simulink model "pam_system"  (R2024b)
settings: Solver=VariableStepAuto  StartTime=0.0  StopTime=1  RelTol=1e-3
model workspace (MAT data in the model file):
  bit_interval = 0.01
  carrier_interval = 0.001
  reference_energy = 0.005
  sampling_interval = 0.0001
undefined symbols (not defined in the file or in its folder): DiscIntNeverNeededParam
libraries: commchan3 x1, commrandsrc3 x1
settings Model: Creator=YN53IX  LastModifiedBy=rasm2
settings SolverCC: AlgebraicLoopSolver=TrustRegion
settings DebuggingCC: ArithmeticOperatorsInVariantConditions=warning
settings SFSimCC: CustomCodeUndefinedFunction=UseInterfaceOnly
settings RTWCC: GPUComputeCapability=3.5

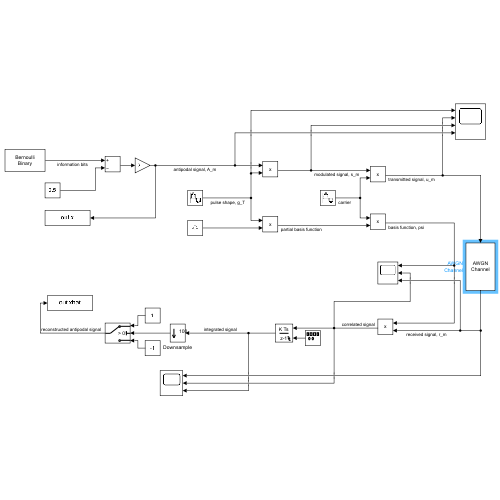
[thumbnail: Simulink's stored preview of the top-level diagram]
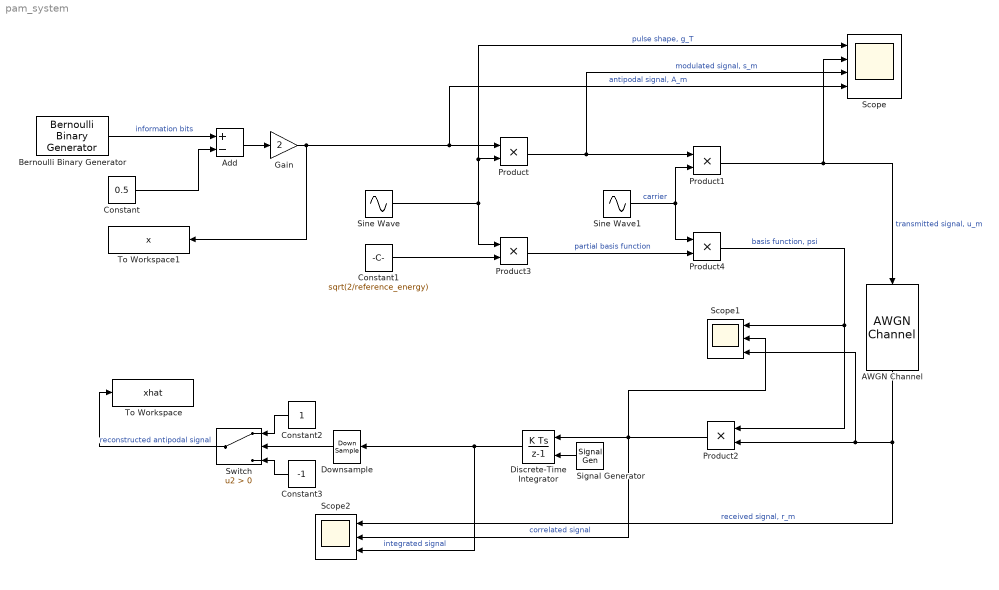
== system pam_system ==
  AWGN Channel : commchan3/AWGN Channel  LegacyMode=on  NoiseMethod="Signal to noise ratio  (SNR)"  noiseMode="Signal to noise ratio  (SNR)"  EbNo=0  EsNo=10  SNR=-10  BitsPerSymbol=1  SignalPower=1  SamplesPerSymbol=1  SymbolPeriod=(1.000000e-04 * 1)  VarianceSource=Parameter  Variance=1  RandomStream=Global stream  Seed=42  SimulateUsing=Code generation
  Add : Sum  Inputs=+-
  Bernoulli Binary Generator : commrandsrc3/Bernoulli Binary Generator  ProbabilityOfZero=0.5  SeedSource=Parameter  Seed=42  SampleTime=bit_interval  SamplesPerFrame=1  OutputDataType=double  SimulateUsing=Interpreted execution
  Constant : Constant  Value=0.5
  Constant1 : Constant  Value=sqrt(2/reference_energy)
  Constant2 : Constant
  Constant3 : Constant  Value=-1
  Discrete-Time Integrator : DiscreteIntegrator  ExternalReset=falling  SampleTime=sampling_interval  ICPrevOutput=DiscIntNeverNeededParam  ICPrevScaledInput=DiscIntNeverNeededParam
  Downsample : DownSample  N=100  phase=99  RateOptions=Allow multirate processing
  Gain : Gain  Gain=2
  Product{,1..4} (5 alike) : Product
  Scope : Scope  NumInputPorts=4
  Scope1 : Scope  NumInputPorts=3
  Scope2 : Scope  NumInputPorts=3
  Signal Generator : SignalGenerator  WaveForm=square  Frequency=1/bit_interval
  Sine Wave : Sin  Frequency=2*pi / bit_interval  Phase=pi/2  SampleTime=sampling_interval
  Sine Wave1 : Sin  Frequency=2 * pi / carrier_interval  Phase=pi/2  SampleTime=sampling_interval
  Switch : Switch  Criteria=u2 > Threshold  SaturateOnIntegerOverflow=off  InputSameDT=off
  To Workspace : ToWorkspace  VariableName=xhat  SampleTime=-1
      settings: Save2DSignal=2-D array (concatenate along first dimension)
  To Workspace1 : ToWorkspace  VariableName=x  SampleTime=-1
      settings: Save2DSignal=2-D array (concatenate along first dimension)
  wires:
  Bernoulli Binary Generator/1 -> Add/1  "information bits"
  Constant/1 -> Add/2
  Add/1 -> Gain/1
  Gain/1 -> To Workspace1/1, Scope/4, Product/1  "antipodal signal, A_m"
  Sine Wave/1 -> Scope/1, Product/2, Product3/1  "pulse shape, g_T"
  Product/1 -> Scope/3, Product1/1  "modulated signal, s_m"
  Sine Wave1/1 -> Product1/2, Product4/1  "carrier"
  Product1/1 -> Scope/2, AWGN Channel/1  "transmitted signal, u_m"
  AWGN Channel/1 -> Scope2/1, Scope1/3, Product2/2  "received signal, r_m"
  Product2/1 -> Scope2/2, Scope1/2, Discrete-Time Integrator/1  "correlated signal"
  Constant1/1 -> Product3/2
  Product3/1 -> Product4/2  "partial basis function"
  Product4/1 -> Product2/1, Scope1/1  "basis function, psi"
  Discrete-Time Integrator/1 -> Scope2/3, Downsample/1  "integrated signal"
  Signal Generator/1 -> Discrete-Time Integrator/2
  Constant3/1 -> Switch/3
  Constant2/1 -> Switch/1
  Switch/1 -> To Workspace/1  "reconstructed antipodal signal"
  Downsample/1 -> Switch/2
